simulink library "AE512Blockset"  (R2014a)
settings: Solver=ode45  StartTime=0.0  StopTime=10.0  RelTol=1e-3
undefined symbols (not defined in the file or in its folder): SendPositionOrientationAndCameraViewToXPlaneOverUDP, SendPositionOrientationToXPlaneOverUDP
undefined symbols (not defined in the file): simulation
libraries: aerolibutil x2, vrlib x1, UWAerospaceBlockset_Payloads x1
settings Model: Creator=Christopher  LastModifiedBy=Christopher

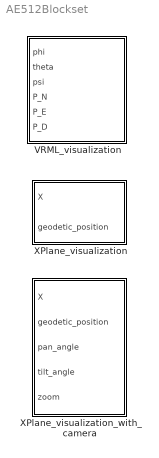
== system AE512Blockset ==
  VRML_visualization : Subsystem
      mask help:
      | Visualize the aircraft using a VRML sink.
      |
      | Note: Simulink should open up the VRML sink and it should display the aircraft model in a separate window.  If this does not occur, you may need to look under the mask and double click on the VR Sink block to open the window.
      |
      | Further note that Simulink may close the VRML sink the first time it is run (it may display a warning with verbiage about 'Virtual world has been closed from outside of Simulink.'.  If this occurs, simply repeat the procedure of looking under the mask and double clicking on the VR Sink.
      |
      | INPUTS: -phi: bank angle (rad)
      |         -theta: pitch angle (rad)
      |         -psi: yaw angle (rad)
      |         -P_N:   position north (m)
      |         -P_E:   position down (m)
      |         -P_D:   position down (m)
      |
      | OUTPUTS: -none
  XPlane_visualization : Subsystem  mask{IP_address=simulation.x_plane.state_visualization.IP_address, plugin_listening_port_number=simulation.x_plane.state_visualization.plugin_listening_port_number, numDigitsOfPrecision=simulation.x_plane.state_visualization.numDigitsOfPrecision}
      mask prompts: IP_address "String of X-Plane machine IP address (i.e. '192.168..112')"; plugin_listening_port_number "Port number that the X-Plane plugin is expecting to receive UDP messages on (i.e. 49003)"; numDigitsOfPrecision "Number of degrees of precision to transmit a string representation of a number over UDP (i.e. 10)"
      mask help:
      | Visualize state of aircraft using X-Plane.
      |
      | The machine running X-Plane should have a plugin operating which disables the internal X-Plane physics engine and listens to state information over UDP (which it then applies to the simulator).
      |
      | INPUT:  -X:   12-by-1 vector of the state [u (m/s);v (m/s);w (m/s);p (rad/s);q (rad/s);r (rad/s);phi (rad);theta (rad);psi (rad);P_N (m);P_E (m);P_D (m)]
      |         -geodetic_position: 3-by-1 vector of [latitude (rad); longitude (rad); altitude (m)]
      |
      | OUTPUT: -none
      |
      | VALIDATION: -unit test
  XPlane_visualization_with_camera : Subsystem  mask{IP_address=simulation.x_plane.camera_visualization.IP_address, plugin_listening_port_number=simulation.x_plane.camera_visualization.plugin_listening_port_number, numDigitsOfPrecision=simulation.x_plane.camera_visualization.numDigitsOfPrecision}
      mask prompts: IP_address "String of X-Plane machine IP address (i.e. '192.47..102')"; plugin_listening_port_number "Port number that the X-Plane plugin is expecting to receive UDP messages on (i.e. 49004)"; numDigitsOfPrecision "Number of degrees of precision to transmit a string representation of a number over UDP (i.e. 10)"
      mask help:
      | Visualize state of aircraft using X-Plane.
      |
      | This includes support for a camera which is located at the same location as the aircraft.
      |
      | The machine running X-Plane should have a plugin operating which disables the internal X-Plane physics engine and listens to state information over UDP (which it then applies to the simulator).
      |
      | INPUT:  -X:             12-by-1 vector of the state [u (m/s);v (m/s);w (m/s);p (rad/s);q (rad/s);r (rad/s);phi (rad);theta (rad);psi (rad);P_N (m);P_E (m);P_D (m)]
      |         -geodetic_position: 3-by-1 vector of [latitude (rad); longitude (rad); altitude (m)]
      |         -pan_angle:     pan angle of camera (rad)
      |         -tilt_angle:    tilt angle of camera (rad)
      |         -zoom:          zoom factor (1 = no zoom, 2 = double zoom)
      |
      | OUTPUT: -none
      |
      | VALIDATION: -unit test

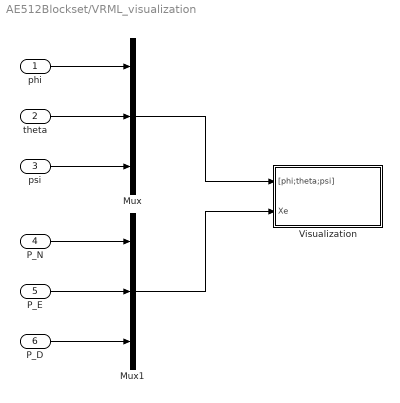
== system AE512Blockset/VRML_visualization ==
  phi : Inport
  theta : Inport  Port=2
  psi : Inport  Port=3
  P_N : Inport  Port=4
  P_E : Inport  Port=5
  P_D : Inport  Port=6
  Mux : Mux  Inputs=3
  Mux1 : Mux  Inputs=3
  Visualization : Subsystem
  wires:
  phi/1 -> Mux/1
  theta/1 -> Mux/2
  psi/1 -> Mux/3
  P_N/1 -> Mux1/1
  P_D/1 -> Mux1/3
  P_E/1 -> Mux1/2
  Mux/1 -> Visualization/1("[phi;theta;psi]")
  Mux1/1 -> Visualization/2(Xe)

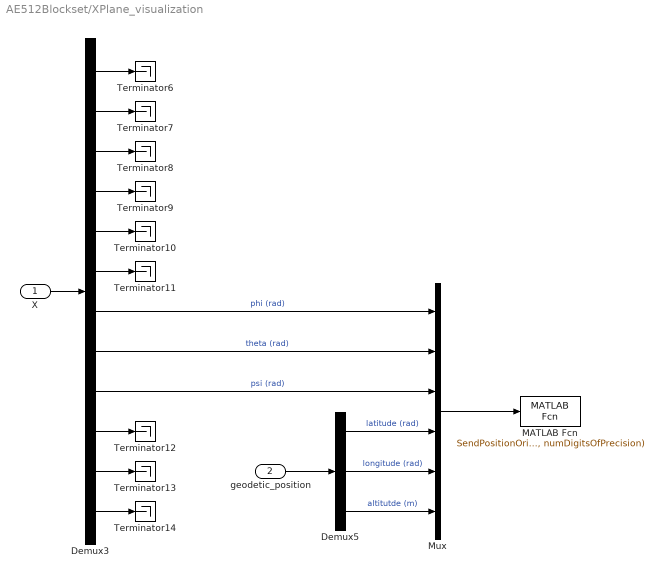
== system AE512Blockset/XPlane_visualization ==
  X : Inport
  geodetic_position : Inport  Port=2
  Demux3 : Demux  Outputs=12
  Demux5 : Demux  Outputs=3
  MATLAB Fcn : MATLABFcn  MATLABFcn=SendPositionOrientationToXPlaneOverUDP(u, IP_address, plugin_listening_port_number, numDigitsOfPrecision)  OutputDimensions=0
  Mux : Mux  Inputs=6
  Terminator{6..14} (9 alike) : Terminator
  wires:
  Mux/1 -> MATLAB Fcn/1
  geodetic_position/1 -> Demux5/1
  X/1 -> Demux3/1
  Demux3/1 -> Terminator6/1
  Demux3/2 -> Terminator7/1
  Demux3/3 -> Terminator8/1
  Demux3/4 -> Terminator9/1
  Demux3/5 -> Terminator10/1
  Demux3/6 -> Terminator11/1
  Demux3/10 -> Terminator12/1
  Demux3/11 -> Terminator13/1
  Demux3/12 -> Terminator14/1
  Demux3/7 -> Mux/1  "phi (rad)"
  Demux3/8 -> Mux/2  "theta (rad)"
  Demux3/9 -> Mux/3  "psi (rad)"
  Demux5/1 -> Mux/4  "latitude (rad)"
  Demux5/2 -> Mux/5  "longitude (rad)"
  Demux5/3 -> Mux/6  "altitutde (m)"

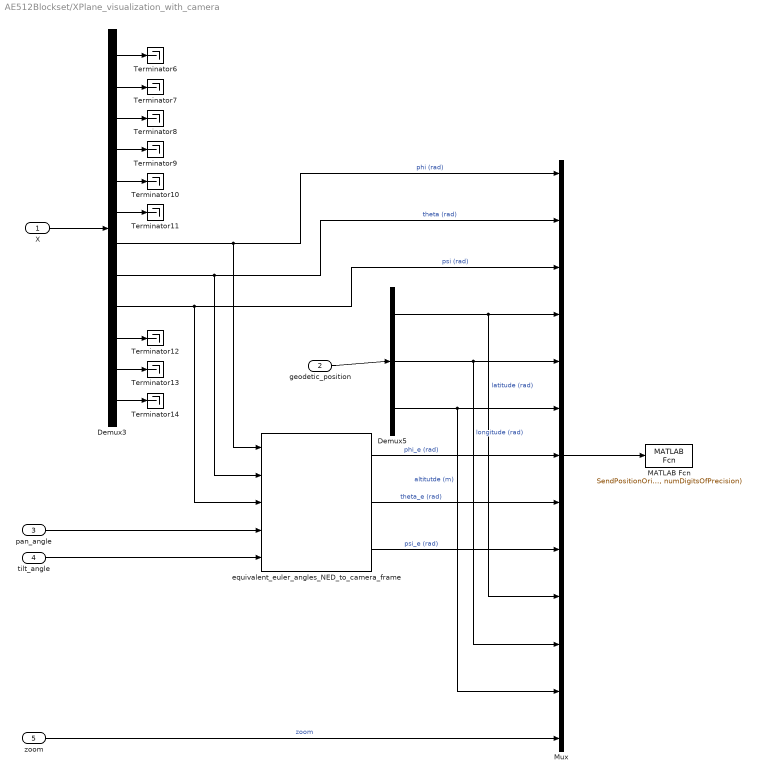
== system AE512Blockset/XPlane_visualization_with_camera ==
  X : Inport
  geodetic_position : Inport  Port=2
  pan_angle : Inport  Port=3
  tilt_angle : Inport  Port=4
  zoom : Inport  Port=5
  Demux3 : Demux  Outputs=12
  Demux5 : Demux  Outputs=3
  MATLAB Fcn : MATLABFcn  MATLABFcn=SendPositionOrientationAndCameraViewToXPlaneOverUDP(u, IP_address, plugin_listening_port_number, numDigitsOfPrecision)  OutputDimensions=0
  Mux : Mux  Inputs=13
  Terminator{6..14} (9 alike) : Terminator
  equivalent_euler_angles_NED_to_camera_frame : UWAerospaceBlockset_Payloads/equivalent_euler_angles_NED_to_camera_frame
  wires:
  Mux/1 -> MATLAB Fcn/1
  X/1 -> Demux3/1
  pan_angle/1 -> equivalent_euler_angles_NED_to_camera_frame/4
  tilt_angle/1 -> equivalent_euler_angles_NED_to_camera_frame/5
  equivalent_euler_angles_NED_to_camera_frame/1 -> Mux/7  "phi_e (rad)"
  equivalent_euler_angles_NED_to_camera_frame/2 -> Mux/8  "theta_e (rad)"
  equivalent_euler_angles_NED_to_camera_frame/3 -> Mux/9  "psi_e (rad)"
  zoom/1 -> Mux/13  "zoom"
  Demux5/1 -> Mux/4, Mux/10  "latitude (rad)"
  Demux5/3 -> Mux/6, Mux/12  "altitutde (m)"
  geodetic_position/1 -> Demux5/1
  Demux3/1 -> Terminator6/1
  Demux3/2 -> Terminator7/1
  Demux3/3 -> Terminator8/1
  Demux3/4 -> Terminator9/1
  Demux3/5 -> Terminator10/1
  Demux3/6 -> Terminator11/1
  Demux3/10 -> Terminator12/1
  Demux3/11 -> Terminator13/1
  Demux3/12 -> Terminator14/1
  Demux3/7 -> equivalent_euler_angles_NED_to_camera_frame/1, Mux/1  "phi (rad)"
  Demux3/8 -> equivalent_euler_angles_NED_to_camera_frame/2, Mux/2  "theta (rad)"
  Demux3/9 -> equivalent_euler_angles_NED_to_camera_frame/3, Mux/3  "psi (rad)"
  Demux5/2 -> Mux/5, Mux/11  "longitude (rad)"

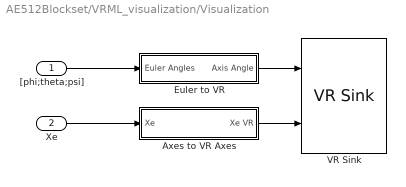
== system AE512Blockset/VRML_visualization/Visualization ==
  "[phi;theta;psi]" : Inport
  Xe : Inport  Port=2
  Axes to VR Axes : Subsystem
  Euler to VR : Subsystem
  VR Sink : vrlib/VR Sink  InstantiateOnLoad=on  SampleTime=-1  ViewEnable=on  RemoteChange=off  RemoteView=off  FieldsWritten=hl20.rotation.4.1.1.double#hl20.translation.3.1.1.double  WorldFileName=aeroblk_HL20.wrl  WorldDescription=aeroblk_HL20  AutoView=on  VideoDimensions=[]  AllowVariableSize=off  FigureProperties="{'Position', 'Name', 'Viewpoint', 'CameraBound', 'CameraDirection', 'CameraPosition', 'CameraUpVector', 'ZoomFactor', 'Antialiasing', 'Headlight', 'Lighting', 'NavPanel', 'StatusBar', 'ToolBar', 'Textures', 'Transparency', 'Triad', 'Wireframe', 'NavZones', 'NavMode', 'NavSpeed', 'CaptureFileFormat', 'CaptureFileName', 'Record2DCompressMethod', 'Record2DCompressQuality', 'Record2D', 'Record2DFileName', 'Record2DFPS'; [5.0000000000000000e+00   9.2000000000000000e+01   5.7600000000000000e+02   3.8000000000000000e+02], 'aeroblk_HL20', 'Fixed Position', 'on', [0.0000000000000000e+00   0.0000000000000000e+00  -1.0000000000000000e+00], [0.0000000000000000e+00   0.0000000000000000e+00   0.0000000000000000e+00], [0.0000000000000000e+00   1.0000000000000000e+00   0.0000000000000000e+00], [1.0000000000000000e+00], 'on', 'on', 'on', 'halfbar', 'on', 'on', 'on', 'on', 'none', 'off', 'off', 'fly', 'normal', 'tif', '%f_anim_%n.tif', 'auto', [7.5000000000000000e+01], 'off', '%f_anim_%n.avi', 'auto'}"
  wires:
  "[phi;theta;psi]"/1 -> Euler to VR/1(Euler Angles)
  Xe/1 -> Axes to VR Axes/1(Xe)
  Axes to VR Axes/1(Xe VR) -> VR Sink/2
  Euler to VR/1(Axis Angle) -> VR Sink/1

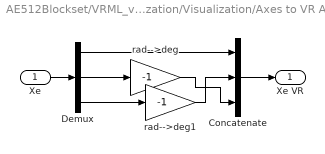
== system AE512Blockset/VRML_visualization/Visualization/Axes to VR Axes ==
  Xe : Inport
  Concatenate : Concatenate  NumInputs=3
  Demux : Demux  Outputs=3
  rad-->deg : Gain  Gain=-1  SaturateOnIntegerOverflow=on  OutDataTypeStr=Inherit: Same as input  ParamDataTypeStr=Inherit: Same as input
  rad-->deg1 : Gain  Gain=-1  SaturateOnIntegerOverflow=on  OutDataTypeStr=Inherit: Same as input  ParamDataTypeStr=Inherit: Same as input
  Xe VR : Outport
  wires:
  Xe/1 -> Demux/1
  Demux/1 -> Concatenate/1
  Demux/2 -> rad-->deg/1
  Demux/3 -> rad-->deg1/1
  Concatenate/1 -> Xe VR/1
  rad-->deg1/1 -> Concatenate/2
  rad-->deg/1 -> Concatenate/3

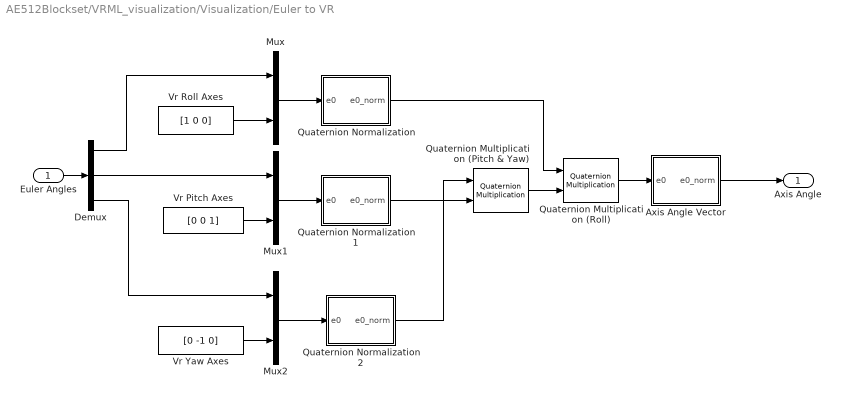
== system AE512Blockset/VRML_visualization/Visualization/Euler to VR ==
  Euler Angles : Inport
  Axis Angle Vector : Subsystem
  Demux : Demux  Outputs=3
  Mux : Mux  Inputs=2
  Mux1 : Mux  Inputs=2
  Mux2 : Mux  Inputs=2
  Quaternion Multiplication (Pitch & Yaw) : aerolibutil/Quaternion Multiplication
  Quaternion Multiplication (Roll) : aerolibutil/Quaternion Multiplication
  Quaternion Normalization : Subsystem
  Quaternion Normalization1 : Subsystem
  Quaternion Normalization2 : Subsystem
  Vr Pitch Axes : Constant  Value=[0 0 1]
  Vr Roll Axes : Constant  Value=[1 0 0]
  Vr Yaw Axes : Constant  Value=[0 -1 0]
  Axis Angle : Outport
  wires:
  Quaternion Multiplication (Roll)/1 -> Axis Angle Vector/1(e0)
  Quaternion Multiplication (Pitch & Yaw)/1 -> Quaternion Multiplication (Roll)/2
  Axis Angle Vector/1(e0_norm) -> Axis Angle/1
  Quaternion Normalization/1(e0_norm) -> Quaternion Multiplication (Roll)/1
  Quaternion Normalization2/1(e0_norm) -> Quaternion Multiplication (Pitch & Yaw)/1
  Quaternion Normalization1/1(e0_norm) -> Quaternion Multiplication (Pitch & Yaw)/2
  Mux2/1 -> Quaternion Normalization2/1(e0)
  Mux1/1 -> Quaternion Normalization1/1(e0)
  Mux/1 -> Quaternion Normalization/1(e0)
  Vr Yaw Axes/1 -> Mux2/2
  Vr Pitch Axes/1 -> Mux1/2
  Vr Roll Axes/1 -> Mux/2
  Euler Angles/1 -> Demux/1
  Demux/1 -> Mux/1
  Demux/2 -> Mux1/1
  Demux/3 -> Mux2/1

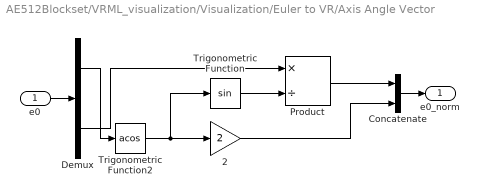
== system AE512Blockset/VRML_visualization/Visualization/Euler to VR/Axis Angle Vector ==
  e0 : Inport
  2 : Gain  Gain=2  SaturateOnIntegerOverflow=on  OutDataTypeStr=Inherit: Same as input  ParamDataTypeStr=Inherit: Same as input
  Concatenate : Concatenate
  Demux : Demux  Outputs=[1 3 ]
  Product : Product  Inputs=*/  SaturateOnIntegerOverflow=on  InputSameDT=on  OutDataTypeStr=Inherit: Same as first input
  Trigonometric Function : Trigonometry
  Trigonometric Function2 : Trigonometry  Operator=acos
  e0_norm : Outport
  wires:
  Demux/1 -> Trigonometric Function2/1
  Demux/2 -> Product/1
  Concatenate/1 -> e0_norm/1
  Product/1 -> Concatenate/1
  2/1 -> Concatenate/2
  Trigonometric Function/1 -> Product/2
  Trigonometric Function2/1 -> Trigonometric Function/1, 2/1
  e0/1 -> Demux/1

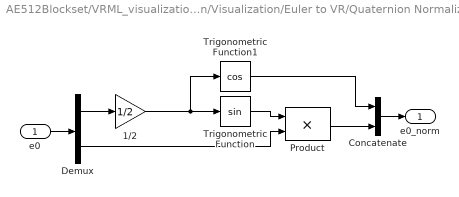
== system AE512Blockset/VRML_visualization/Visualization/Euler to VR/Quaternion Normalization ==
  e0 : Inport
  1/2 : Gain  Gain=1/2  SaturateOnIntegerOverflow=on  OutDataTypeStr=Inherit: Same as input  ParamDataTypeStr=Inherit: Same as input
  Concatenate : Concatenate
  Demux : Demux  Outputs=[1 3]
  Product : Product  SaturateOnIntegerOverflow=on  InputSameDT=on  OutDataTypeStr=Inherit: Same as first input
  Trigonometric Function : Trigonometry
  Trigonometric Function1 : Trigonometry  Operator=cos
  e0_norm : Outport
  wires:
  Trigonometric Function1/1 -> Concatenate/1
  Demux/2 -> Product/2
  Demux/1 -> 1/2/1
  Concatenate/1 -> e0_norm/1
  Product/1 -> Concatenate/2
  Trigonometric Function/1 -> Product/1
  1/2/1 -> Trigonometric Function1/1, Trigonometric Function/1
  e0/1 -> Demux/1

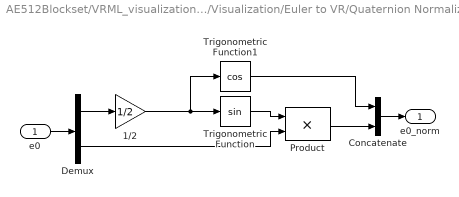
== system AE512Blockset/VRML_visualization/Visualization/Euler to VR/Quaternion Normalization1 ==
  e0 : Inport
  1/2 : Gain  Gain=1/2  SaturateOnIntegerOverflow=on  OutDataTypeStr=Inherit: Same as input  ParamDataTypeStr=Inherit: Same as input
  Concatenate : Concatenate
  Demux : Demux  Outputs=[1 3]
  Product : Product  SaturateOnIntegerOverflow=on  InputSameDT=on  OutDataTypeStr=Inherit: Same as first input
  Trigonometric Function : Trigonometry
  Trigonometric Function1 : Trigonometry  Operator=cos
  e0_norm : Outport
  wires:
  e0/1 -> Demux/1
  1/2/1 -> Trigonometric Function/1, Trigonometric Function1/1
  Trigonometric Function/1 -> Product/1
  Product/1 -> Concatenate/2
  Concatenate/1 -> e0_norm/1
  Demux/1 -> 1/2/1
  Demux/2 -> Product/2
  Trigonometric Function1/1 -> Concatenate/1

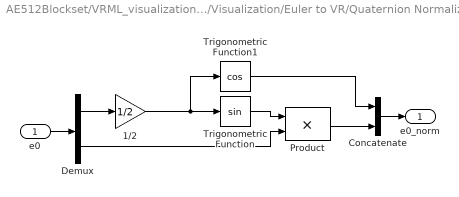
== system AE512Blockset/VRML_visualization/Visualization/Euler to VR/Quaternion Normalization2 ==
  e0 : Inport
  1/2 : Gain  Gain=1/2  SaturateOnIntegerOverflow=on  OutDataTypeStr=Inherit: Same as input  ParamDataTypeStr=Inherit: Same as input
  Concatenate : Concatenate
  Demux : Demux  Outputs=[1 3]
  Product : Product  SaturateOnIntegerOverflow=on  InputSameDT=on  OutDataTypeStr=Inherit: Same as first input
  Trigonometric Function : Trigonometry
  Trigonometric Function1 : Trigonometry  Operator=cos
  e0_norm : Outport
  wires:
  Trigonometric Function1/1 -> Concatenate/1
  Demux/2 -> Product/2
  Demux/1 -> 1/2/1
  Concatenate/1 -> e0_norm/1
  Product/1 -> Concatenate/2
  Trigonometric Function/1 -> Product/1
  1/2/1 -> Trigonometric Function1/1, Trigonometric Function/1
  e0/1 -> Demux/1
